simulink model "Microspeaker"  (R2024a)
settings: Solver=daessc  StartTime=0.0  StopTime=T  MaxStep=1/441000  RelTol=1e-3  AbsTol=1e-3
model workspace (MAT data in the model file):
  T = Simulink.Parameter
  T.Value = 3
  T.Complexity = 'real'
  T.Dimensions = [1 1]
  T.Description = 'simulation time '
  T.DataType = 'auto'
  dt = Simulink.Parameter
  dt.Value = 2.26757369615e-05
  dt.Complexity = 'real'
  dt.Dimensions = [1 1]
  dt.Description = 'sampling time '
  dt.DataType = 'auto'
libraries: acoustic_lib x14, fl_lib x13, nesl_utility x7, simulink x1
settings Model: Creator=andychen  LastModifiedBy=ftiong
settings DataIOCC: OutputOption=SpecifiedOutputTimes  OutputTimes=0:dt:T

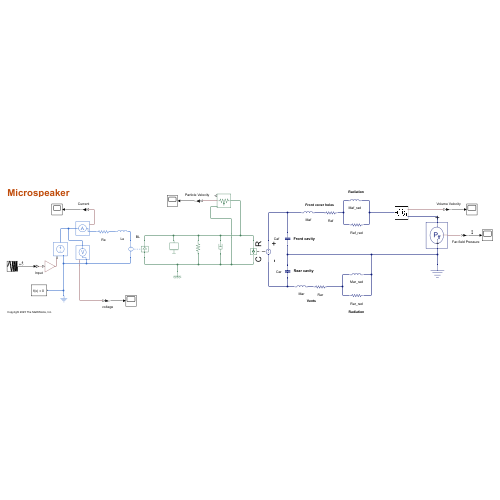
[thumbnail: Simulink's stored preview of the top-level diagram]
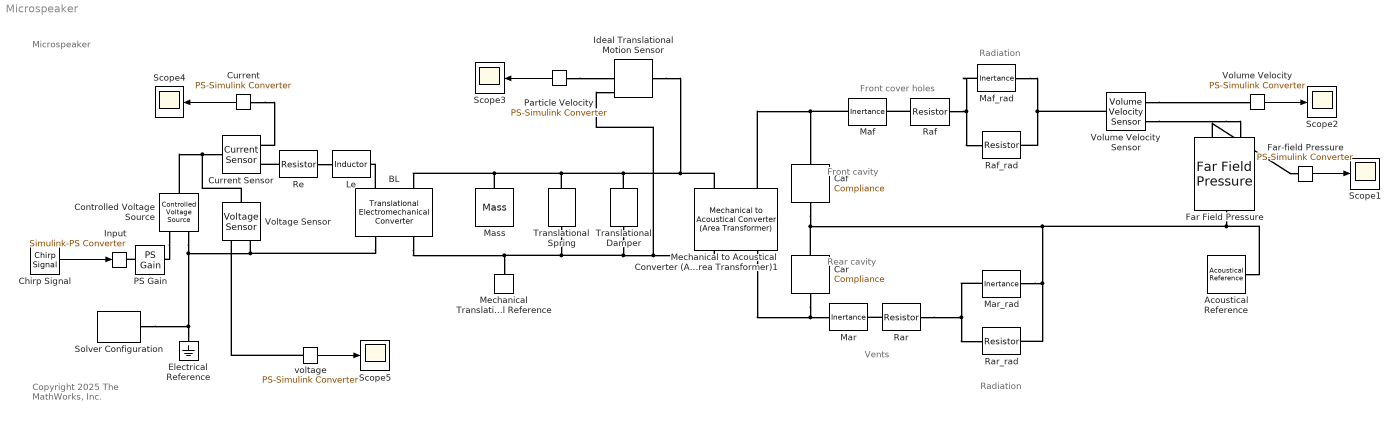
== system Microspeaker ==
  note: Front cavity
  note: Radiation
  note: Front cover holes
  note: Vents
  note: Radiation
  note: Microspeaker
  note: Rear cavity
  note: Copyright 2025 The MathWorks, Inc.
  Acoustical Reference : acoustic_lib/Acoustical Elements/Acoustical Reference
      settings: SourceProductName=Acoustic  InternalSimscapePortConfiguration="{\"Bottom\":[],\"Left\":[],\"Right\":[],\"Top\":[{\"id\":\"pp\",\"label\":\"\",\"type\":\"acoustic.acoustic\"}]}"
  BL : fl_lib/Electrical/Electrical Elements/Translational Electromechanical Converter  K=0.719 V*s/m  i_specify=off  i_priority=None  i=0 A  i_nominal_specify=off  i_nominal_value=1  i_nominal_unit=A  v_specify=off  v_priority=None  v=0 V  v_nominal_specify=off  v_nominal_value=1  v_nominal_unit=V  f_specify=off  f_priority=None  f=0 N  f_nominal_specify=off  f_nominal_value=1  f_nominal_unit=N  u_specify=off  u_priority=None  u=0 m/s  u_nominal_specify=off  u_nominal_value=1  u_nominal_unit=m/s
      settings: InternalSimscapePortConfiguration="{\"Bottom\":[],\"Left\":[{\"id\":\"p\",\"label\":\"+\",\"type\":\"foundation.electrical.electrical\"},{\"id\":\"R\",\"label\":\"R\",\"type\":\"foundation.mechanical.translational.translational\"}],\"Right\":[{\"id\":\"n\",\"label\":\"-\",\"type\":\"foundation.electrical.electrical\"},{\"id\":\"C\",\"label\":\"C\",\"type\":\"foundation.mechanical.translational.translational\"}],\"Top\":[]}"
  Caf : acoustic_lib/Acoustical Elements/Compliance  c=7.197e-13 m^3/Pa  r_c=0 Pa*s/m^3  g_c=0 m^3/(Pa*s)  u_specify=off  u_priority=None  u=0 m^3/s  u_nominal_specify=off  u_nominal_value=1  u_nominal_unit=m^3/s  p_specify=off  p_priority=None  p=0 Pa  p_nominal_specify=off  p_nominal_value=1  p_nominal_unit=Pa  Pc_specify=off  Pc_priority=High  Pc=0 Pa  Pc_nominal_specify=off  Pc_nominal_value=1  Pc_nominal_unit=Pa
      settings: SourceProductName=Acoustic  InternalSimscapePortConfiguration="{\"Bottom\":[],\"Left\":[{\"id\":\"pp\",\"label\":\"+\",\"type\":\"acoustic.acoustic\"}],\"Right\":[{\"id\":\"nn\",\"label\":\"-\",\"type\":\"acoustic.acoustic\"}],\"Top\":[]}"
  Car : acoustic_lib/Acoustical Elements/Compliance  c=7.1403e-13 m^3/Pa  r_c=0 Pa*s/m^3  g_c=0 m^3/(Pa*s)  u_specify=off  u_priority=None  u=0 m^3/s  u_nominal_specify=off  u_nominal_value=1  u_nominal_unit=m^3/s  p_specify=off  p_priority=None  p=0 Pa  p_nominal_specify=off  p_nominal_value=1  p_nominal_unit=Pa  Pc_specify=off  Pc_priority=High  Pc=0 Pa  Pc_nominal_specify=off  Pc_nominal_value=1  Pc_nominal_unit=Pa
      settings: SourceProductName=Acoustic  InternalSimscapePortConfiguration="{\"Bottom\":[],\"Left\":[{\"id\":\"pp\",\"label\":\"+\",\"type\":\"acoustic.acoustic\"}],\"Right\":[{\"id\":\"nn\",\"label\":\"-\",\"type\":\"acoustic.acoustic\"}],\"Top\":[]}"
  Chirp Signal : simulink/Sources/Chirp Signal  f1=10  T=T  f2=20e3
  Controlled Voltage Source : fl_lib/Electrical/Electrical Sources/Controlled Voltage Source
  Current : nesl_utility/PS-Simulink Converter  PhysicalDomain=network_engine_domain  SubClassName=ps_output  LeftPortType=input  RightPortType=output  PseudoPeriodic=off  Frequencies=[]  VectorFormat=inherit  Unit=inherit  AffineConversion=off
  Current Sensor : fl_lib/Electrical/Electrical Sensors/Current Sensor
  Electrical Reference : fl_lib/Electrical/Electrical Elements/Electrical Reference
  Far Field Pressure : acoustic_lib/Acoustical Sensors/Far Field Pressure  dist=10 cm  u_specify=off  u_priority=None  u=0 m^3/s  u_nominal_specify=off  u_nominal_value=1  u_nominal_unit=m^3/s  p_specify=off  p_priority=None  p=0 Pa  p_nominal_specify=off  p_nominal_value=1  p_nominal_unit=Pa
      settings: SourceProductName=Acoustic  InternalSimscapePortConfiguration="{\"Bottom\":[],\"Left\":[{\"id\":\"pp\",\"label\":\"+\",\"type\":\"acoustic.acoustic\"}],\"Right\":[{\"id\":\"nn\",\"label\":\"-\",\"type\":\"acoustic.acoustic\"}],\"Top\":[{\"id\":\"p_ff\",\"label\":\"\",\"type\":\"output\"}]}"
  Far-field Pressure : nesl_utility/PS-Simulink Converter  PhysicalDomain=network_engine_domain  SubClassName=ps_output  LeftPortType=input  RightPortType=output  PseudoPeriodic=off  Frequencies=[]  VectorFormat=inherit  Unit=inherit  AffineConversion=off
  Ideal Translational Motion Sensor : fl_lib/Mechanical/Mechanical Sensors/Ideal Translational Motion Sensor  reference=foundation.enum.MeasurementReference.difference  acceleration_port=false  velocity_port=true  position_port=true  offset=0 m
  Input : nesl_utility/Simulink-PS Converter  PhysicalDomain=network_engine_domain  SubClassName=ps_input  LeftPortType=input  RightPortType=output  PseudoPeriodic=off  Frequencies=[]  NoiseDistribution=none  NoiseParameters=[]  Unit=1  AffineConversion=off  FilteringAndDerivatives=provide  SimscapeFilterOrder=1  InputFilterTimeConstant=0.001  UdotUserProvided=0
  Le : fl_lib/Electrical/Electrical Elements/Inductor  l=14e-5 H  r=0 Ohm  g=1e-9 1/Ohm  i_specify=off  i_priority=None  i=0 A  i_nominal_specify=off  i_nominal_value=1  i_nominal_unit=A  v_specify=off  v_priority=None  v=0 V  v_nominal_specify=off  v_nominal_value=1  v_nominal_unit=V  i_L_specify=off  i_L_priority=High  i_L=0 A  i_L_nominal_specify=off  i_L_nominal_value=1  i_L_nominal_unit=A
  Maf : acoustic_lib/Acoustical Elements/Inertance  m=17.118 Pa*s^2/m^3  r_m=1e-9 Pa*s/m^3  g_m=1e-9 m^3/(Pa*s)  u_specify=off  u_priority=None  u=0 m^3/s  u_nominal_specify=off  u_nominal_value=1  u_nominal_unit=m^3/s  p_specify=off  p_priority=None  p=0 Pa  p_nominal_specify=off  p_nominal_value=1  p_nominal_unit=Pa  U_m_specify=off  U_m_priority=High  U_m=0 m^3/s  U_m_nominal_specify=off  U_m_nominal_value=1  U_m_nominal_unit=m^3/s
      settings: SourceProductName=Acoustic  InternalSimscapePortConfiguration="{\"Bottom\":[],\"Left\":[{\"id\":\"pp\",\"label\":\"+\",\"type\":\"acoustic.acoustic\"}],\"Right\":[{\"id\":\"nn\",\"label\":\"-\",\"type\":\"acoustic.acoustic\"}],\"Top\":[]}"
  Maf_rad : acoustic_lib/Acoustical Elements/Inertance  m=104.86 Pa*s^2/m^3  r_m=1e-9 Pa*s/m^3  g_m=1e-9 m^3/(Pa*s)  u_specify=off  u_priority=None  u=0 m^3/s  u_nominal_specify=off  u_nominal_value=1  u_nominal_unit=m^3/s  p_specify=off  p_priority=None  p=0 Pa  p_nominal_specify=off  p_nominal_value=1  p_nominal_unit=Pa  U_m_specify=off  U_m_priority=High  U_m=0 m^3/s  U_m_nominal_specify=off  U_m_nominal_value=1  U_m_nominal_unit=m^3/s
      settings: SourceProductName=Acoustic  InternalSimscapePortConfiguration="{\"Bottom\":[],\"Left\":[{\"id\":\"pp\",\"label\":\"+\",\"type\":\"acoustic.acoustic\"}],\"Right\":[{\"id\":\"nn\",\"label\":\"-\",\"type\":\"acoustic.acoustic\"}],\"Top\":[]}"
  Mar : acoustic_lib/Acoustical Elements/Inertance  m=190.94 Pa*s^2/m^3  r_m=1e-9 Pa*s/m^3  g_m=1e-9 m^3/(Pa*s)  u_specify=off  u_priority=None  u=0 m^3/s  u_nominal_specify=off  u_nominal_value=1  u_nominal_unit=m^3/s  p_specify=off  p_priority=None  p=0 Pa  p_nominal_specify=off  p_nominal_value=1  p_nominal_unit=Pa  U_m_specify=off  U_m_priority=High  U_m=0 m^3/s  U_m_nominal_specify=off  U_m_nominal_value=1  U_m_nominal_unit=m^3/s
      settings: SourceProductName=Acoustic  InternalSimscapePortConfiguration="{\"Bottom\":[],\"Left\":[{\"id\":\"pp\",\"label\":\"+\",\"type\":\"acoustic.acoustic\"}],\"Right\":[{\"id\":\"nn\",\"label\":\"-\",\"type\":\"acoustic.acoustic\"}],\"Top\":[]}"
  Mar_rad : acoustic_lib/Acoustical Elements/Inertance  m=87.46 Pa*s^2/m^3  r_m=1e-9 Pa*s/m^3  g_m=1e-9 m^3/(Pa*s)  u_specify=off  u_priority=None  u=0 m^3/s  u_nominal_specify=off  u_nominal_value=1  u_nominal_unit=m^3/s  p_specify=off  p_priority=None  p=0 Pa  p_nominal_specify=off  p_nominal_value=1  p_nominal_unit=Pa  U_m_specify=off  U_m_priority=High  U_m=0 m^3/s  U_m_nominal_specify=off  U_m_nominal_value=1  U_m_nominal_unit=m^3/s
      settings: SourceProductName=Acoustic  InternalSimscapePortConfiguration="{\"Bottom\":[],\"Left\":[{\"id\":\"pp\",\"label\":\"+\",\"type\":\"acoustic.acoustic\"}],\"Right\":[{\"id\":\"nn\",\"label\":\"-\",\"type\":\"acoustic.acoustic\"}],\"Top\":[]}"
  Mass : fl_lib/Mechanical/Translational Elements/Mass  mass=23e-6 kg  num_ports=foundation.enum.numPorts2.one  v_specify=off  v_priority=High  v=0 m/s  v_nominal_specify=off  v_nominal_value=1  v_nominal_unit=m/s  f_specify=off  f_priority=None  f=0 N  f_nominal_specify=off  f_nominal_value=1  f_nominal_unit=N
  Mechanical Translational Reference : fl_lib/Mechanical/Translational Elements/Mechanical Translational Reference
  Mechanical to Acoustical Converter (Area Transformer)1 : acoustic_lib/Transformers/Mechanical to Acoustical Converter (Area Transformer)  Sd=(18.95e-3/2)^2*pi m^2  u_specify=off  u_priority=None  u=0 m^3/s  u_nominal_specify=off  u_nominal_value=1  u_nominal_unit=m^3/s  p_specify=off  p_priority=None  p=0 Pa  p_nominal_specify=off  p_nominal_value=1  p_nominal_unit=Pa  f_specify=off  f_priority=None  f=0 N  f_nominal_specify=off  f_nominal_value=1  f_nominal_unit=N  v_specify=off  v_priority=None  v=0 m/s  v_nominal_specify=off  v_nominal_value=1  v_nominal_unit=m/s
      settings: SourceProductName=Acoustic  InternalSimscapePortConfiguration="{\"Bottom\":[],\"Left\":[{\"id\":\"pp\",\"label\":\"+\",\"type\":\"acoustic.acoustic\"},{\"id\":\"R\",\"label\":\"R\",\"type\":\"foundation.mechanical.translational.translational\"}],\"Right\":[{\"id\":\"nn\",\"label\":\"-\",\"type\":\"acoustic.acoustic\"},{\"id\":\"C\",\"label\":\"C\",\"type\":\"foundation.mechanical.translational.translational\"}],\"Top\":[]}"
  PS Gain : fl_lib/Physical Signals/Functions/PS Gain  gain=0.179 V
  Particle Velocity : nesl_utility/PS-Simulink Converter  PhysicalDomain=network_engine_domain  SubClassName=ps_output  LeftPortType=input  RightPortType=output  PseudoPeriodic=off  Frequencies=[]  VectorFormat=inherit  Unit=inherit  AffineConversion=off
  Raf : acoustic_lib/Acoustical Elements/Resistor  R_r=6145.5 Pa*s/m^3  u_specify=off  u_priority=None  u=0 m^3/s  u_nominal_specify=off  u_nominal_value=1  u_nominal_unit=m^3/s  p_specify=off  p_priority=None  p=0 Pa  p_nominal_specify=off  p_nominal_value=1  p_nominal_unit=Pa
      settings: SourceProductName=Acoustic  InternalSimscapePortConfiguration="{\"Bottom\":[],\"Left\":[{\"id\":\"pp\",\"label\":\"+\",\"type\":\"acoustic.acoustic\"}],\"Right\":[{\"id\":\"nn\",\"label\":\"-\",\"type\":\"acoustic.acoustic\"}],\"Top\":[]}"
  Raf_rad : acoustic_lib/Acoustical Elements/Resistor  R_r=19.47e6 Pa*s/m^3  u_specify=off  u_priority=None  u=0 m^3/s  u_nominal_specify=off  u_nominal_value=1  u_nominal_unit=m^3/s  p_specify=off  p_priority=None  p=0 Pa  p_nominal_specify=off  p_nominal_value=1  p_nominal_unit=Pa
      settings: SourceProductName=Acoustic  InternalSimscapePortConfiguration="{\"Bottom\":[],\"Left\":[{\"id\":\"pp\",\"label\":\"+\",\"type\":\"acoustic.acoustic\"}],\"Right\":[{\"id\":\"nn\",\"label\":\"-\",\"type\":\"acoustic.acoustic\"}],\"Top\":[]}"
  Rar : acoustic_lib/Acoustical Elements/Resistor  R_r=1.0194e+05 Pa*s/m^3  u_specify=off  u_priority=None  u=0 m^3/s  u_nominal_specify=off  u_nominal_value=1  u_nominal_unit=m^3/s  p_specify=off  p_priority=None  p=0 Pa  p_nominal_specify=off  p_nominal_value=1  p_nominal_unit=Pa
      settings: SourceProductName=Acoustic  InternalSimscapePortConfiguration="{\"Bottom\":[],\"Left\":[{\"id\":\"pp\",\"label\":\"+\",\"type\":\"acoustic.acoustic\"}],\"Right\":[{\"id\":\"nn\",\"label\":\"-\",\"type\":\"acoustic.acoustic\"}],\"Top\":[]}"
  Rar_rad : acoustic_lib/Acoustical Elements/Resistor  R_r=13.59e6 Pa*s/m^3  u_specify=off  u_priority=None  u=0 m^3/s  u_nominal_specify=off  u_nominal_value=1  u_nominal_unit=m^3/s  p_specify=off  p_priority=None  p=0 Pa  p_nominal_specify=off  p_nominal_value=1  p_nominal_unit=Pa
      settings: SourceProductName=Acoustic  InternalSimscapePortConfiguration="{\"Bottom\":[],\"Left\":[{\"id\":\"pp\",\"label\":\"+\",\"type\":\"acoustic.acoustic\"}],\"Right\":[{\"id\":\"nn\",\"label\":\"-\",\"type\":\"acoustic.acoustic\"}],\"Top\":[]}"
  Re : fl_lib/Electrical/Electrical Elements/Resistor  R=31.14 Ohm  i_specify=off  i_priority=None  i=0 A  i_nominal_specify=off  i_nominal_value=1  i_nominal_unit=A  v_specify=off  v_priority=None  v=0 V  v_nominal_specify=off  v_nominal_value=1  v_nominal_unit=V
  Scope{1..5} (5 alike) : Scope
  Solver Configuration : nesl_utility/Solver Configuration  PhysicalDomain=network_engine_domain  SubClassName=solver  LeftPortType=input  RightPortType=generic  Tones=[]  Harmonics=[]  SimulateNoise=off  Profile=off  UseLocalSampling=off  EnableSwitchedLinearOptims=on  FrequencyDomain=off  UseCCode=off  RelTol=0.001  AbsTol=0.001  MinStep=1e-09  ToWorkspace=off  RevertToSquareIcSolve=off  NumHomotopyIterations=100  PhasorMode=off  PhasorModeNumHarmonics=1  ConsistencySolver=NEWTON_XTOL_AFTER_FTOL  IndexReductionMethod=DerivativeReplacement  DoDC=off  ResidualTolerance=1e-09  ConsistencyTolSource=GLOBAL  ConsistencyAbsTol=0.001  ConsistencyRelTol=0.001  ConsistencyTolFactor=0.001  UseLocalSolver=off  LocalSolverChoice=NE_BACKWARD_EULER_ADVANCER  ResolveIndetEquations=on  FunctionEvalNumThread=1  LocalSolverSampleTime=0.001  DoFixedCost=off  MaxNonlinIter=3  MaxModeIter=2  ComputeImpulses=off  ImpulseIterations=2  LinearAlgebra=auto  LinearAlgebraNumThread=0  EquationFormulation=NE_TIME_EF  DelaysMemoryBudget=1024  AutomaticFiltering=on  FilteringTimeConstant=0.001  PartitionStorageMethod=AS_NEEDED  PartitionMemoryBudget=1024  PartitionMethod=ROBUST  MultibodyUseLocalSolver=off  MultibodyLocalSolverChoice=ODE1  MultibodyLocalSolverSampleTime=0.001
  Translational Damper : fl_lib/Mechanical/Translational Elements/Translational Damper  D=3e-3 kg/s  v_specify=off  v_priority=None  v=0 m/s  v_nominal_specify=off  v_nominal_value=1  v_nominal_unit=m/s  f_specify=off  f_priority=None  f=0 N  f_nominal_specify=off  f_nominal_value=1  f_nominal_unit=N
  Translational Spring : fl_lib/Mechanical/Translational Elements/Translational Spring  spr_rate=1 / (25.12e-3) N/m  v_specify=off  v_priority=None  v=0 m/s  v_nominal_specify=off  v_nominal_value=1  v_nominal_unit=m/s  f_specify=off  f_priority=None  f=0 N  f_nominal_specify=off  f_nominal_value=1  f_nominal_unit=N  x_specify=off  x_priority=High  x=0 m  x_nominal_specify=off  x_nominal_value=1  x_nominal_unit=m
  Voltage Sensor : fl_lib/Electrical/Electrical Sensors/Voltage Sensor
  Volume Velocity : nesl_utility/PS-Simulink Converter  PhysicalDomain=network_engine_domain  SubClassName=ps_output  LeftPortType=input  RightPortType=output  PseudoPeriodic=off  Frequencies=[]  VectorFormat=inherit  Unit=inherit  AffineConversion=off
  Volume Velocity Sensor : acoustic_lib/Acoustical Sensors/Volume Velocity Sensor
      settings: SourceProductName=Acoustic  InternalSimscapePortConfiguration="{\"Bottom\":[],\"Left\":[{\"id\":\"pp\",\"label\":\"+\",\"type\":\"acoustic.acoustic\"}],\"Right\":[{\"id\":\"u\",\"label\":\"I\",\"type\":\"output\"},{\"id\":\"nn\",\"label\":\"-\",\"type\":\"acoustic.acoustic\"}],\"Top\":[]}"
  voltage : nesl_utility/PS-Simulink Converter  PhysicalDomain=network_engine_domain  SubClassName=ps_output  LeftPortType=input  RightPortType=output  PseudoPeriodic=off  Frequencies=[]  VectorFormat=inherit  Unit=inherit  AffineConversion=off
  wires:
  Current/1 -> Scope4/1
  Particle Velocity/1 -> Scope3/1
  Far-field Pressure/1 -> Scope1/1
  voltage/1 -> Scope5/1
  Volume Velocity/1 -> Scope2/1
  Chirp Signal/1 -> Input/1
  connections:
  Translational Spring/RConn1 -- BL/RConn2 -- Mechanical Translational Reference/LConn1 -- Mechanical to Acoustical Converter (Area Transformer)1/RConn2 -- Ideal Translational Motion Sensor/RConn1 -- Translational Damper/RConn1
  Mechanical to Acoustical Converter (Area Transformer)1/LConn2 -- Ideal Translational Motion Sensor/LConn1 -- Mass/LConn1 -- BL/LConn2 -- Translational Spring/LConn1 -- Translational Damper/LConn1
  Voltage Sensor/LConn1 -- Controlled Voltage Source/LConn1 -- Current Sensor/LConn1
  Current/LConn1 -- Current Sensor/RConn1
  Controlled Voltage Source/RConn1 -- PS Gain/RConn1
  Particle Velocity/LConn1 -- Ideal Translational Motion Sensor/RConn2
  PS Gain/LConn1 -- Input/RConn1
  voltage/LConn1 -- Voltage Sensor/RConn1
  BL/LConn1 -- Le/RConn1
  Re/RConn1 -- Le/LConn1
  Raf/LConn1 -- Maf/RConn1
  Maf_rad/LConn1 -- Raf_rad/LConn1 -- Raf/RConn1
  Car/RConn1 -- Acoustical Reference/LConn1 -- Far Field Pressure/RConn1 -- Rar_rad/RConn1 -- Mar_rad/RConn1 -- Caf/RConn1
  Car/LConn1 -- Mechanical to Acoustical Converter (Area Transformer)1/RConn1 -- Mar/LConn1
  Rar/LConn1 -- Mar/RConn1
  Maf_rad/RConn1 -- Volume Velocity Sensor/LConn1 -- Raf_rad/RConn1
  Mar_rad/LConn1 -- Rar/RConn1 -- Rar_rad/LConn1
  Maf/LConn1 -- Mechanical to Acoustical Converter (Area Transformer)1/LConn1 -- Caf/LConn1
  Volume Velocity Sensor/RConn1 -- Volume Velocity/LConn1
  Solver Configuration/RConn1 -- Controlled Voltage Source/RConn2 -- BL/RConn1 -- Voltage Sensor/RConn2 -- Electrical Reference/LConn1
  Far Field Pressure/LConn2 -- Far-field Pressure/LConn1
  Volume Velocity Sensor/RConn2 -- Far Field Pressure/LConn1
  Re/LConn1 -- Current Sensor/RConn2
